simulink model "Lab1"  (R2023b)
settings: Solver=VariableStepAuto  StartTime=0.0  StopTime=10  RelTol=1e-3
undefined symbols (not defined in the file): sigbuilder_block
libraries: fl_lib x35, sh_lib x22, nesl_utility x20
settings Model: Creator=agluh  LastModifiedBy=a2
settings SolverCC: AlgebraicLoopSolver=TrustRegion
settings ModelReferenceCC: EnableRefExpFcnMdlSchedulingChecks=on
settings SimscapeCC: ExplicitSolverDiagnosticOptions=none

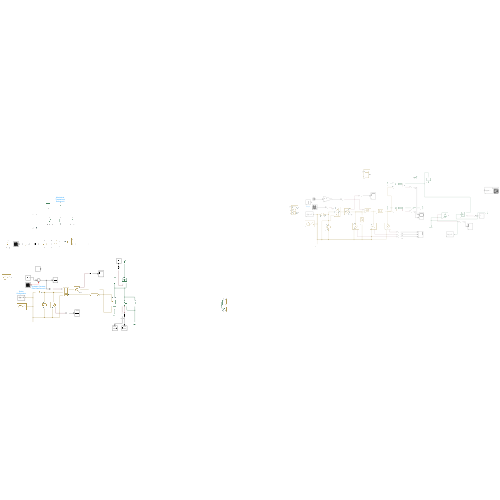
[thumbnail: Simulink's stored preview of the top-level diagram]
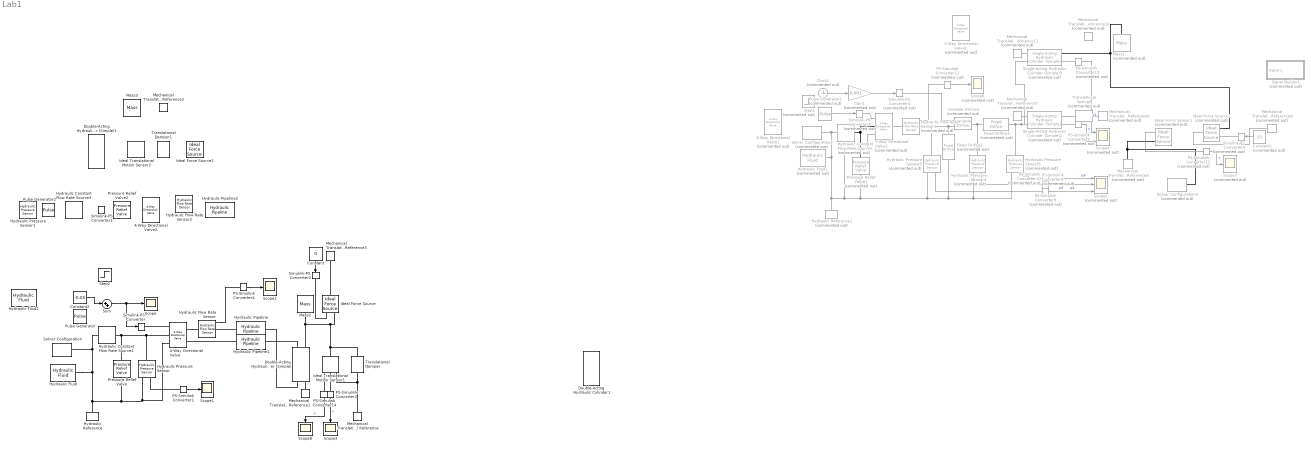
== system Lab1 ==
  2-Way Directional Valve2 : sh_lib/Valves/Directional Valves/2-Way Directional Valve  Commented=on  mdl_type=1  area_max=0.1 m^2  opening_max=0.1 m  opening_tab=[-.002, 0, .002, .005, .015] m  area_tab=[1e-09, 2.0352e-07, 4.0736e-05, .00011438, .00034356] m^2  pressure_tab=[-10000000, -5000000, -2000000, 2000000, 5000000, 10000000] Pa  flow_rate_tab=[-1e-07, -7.0711e-08, -4.4721e-08, 4.4721e-08, 7.0711e-08, 1e-07; -2.0352e-05, -1.4391e-05, -9.1017e-06, 9.1017e-06, 1.4391e-05, 2.0352e-05; -.0040736, -.0028805, -.0018218, .0018218, .0028805, .0040736; -.011438, -.0080879, -.0051152, .0051152, .0080879, .011438; -.034356, -.024293, -.015364, .015364, .024293, .034356] m^3/s  interp_method=1  extrap_method=1  C_d=0.7  x_0=0 m  A_leak=1e-12 m^2  lam_spec=1  B_lam=0.999  Re_cr=12
      settings: InternalSimscapePortConfiguration="{\"Bottom\":[],\"Left\":[{\"id\":\"S\",\"label\":\"S\",\"type\":\"input\"},{\"id\":\"A\",\"label\":\"A\",\"type\":\"foundation.hydraulic.hydraulic\"}],\"Right\":[{\"id\":\"B\",\"label\":\"B\",\"type\":\"foundation.hydraulic.hydraulic\"}],\"Top\":[]}"
  3-Way Directional Valve1 : sh_lib/Valves/Directional Valves/3-Way Directional Valve  Commented=on  area_spec=sh.valves.directional_valves.enum.area_spec.identical  mdl_type_identical=sh.valves.directional_valves.enum.mdl_type.linear  mdl_type_different=sh.valves.directional_valves.enum.mdl_type.linear  interp_method_identical=sh.valves.directional_valves.enum.interp_method.linear  interp_method_different=sh.valves.directional_valves.enum.interp_method.linear  extrap_method_identical=sh.valves.directional_valves.enum.extrap_method.linear  extrap_method_different=sh.valves.directional_valves.enum.extrap_method.linear  A_leak=0.0000000000001 mm^2  C_d=0.7  lam_spec=sh.valves.directional_valves.enum.lam_spec.pressure_ratio  B_lam=0.999  Re_cr=12  opening_max=0.1 m  area_max=0.1 m^2  opening_max_P_A=0.005 m  area_max_P_A=0.5e-4 m^2  opening_max_A_T=0.005 m  area_max_A_T=0.5e-4 m^2  opening_area_tab=[-.002, 0, .002, .005, .015] m  area_tab=[1e-09, 2.0352e-07, 4.0736e-05, .00011438, .00034356] m^2  opening_flow_rate_tab=[-.002, 0, .002, .005, .015] m  pressure_tab=[-10000000, -5000000, -2000000, 2000000, 5000000, 10000000] Pa  flow_rate_tab=[-1e-07, -7.0711e-08, -4.4721e-08, 4.4721e-08, 7.0711e-08, 1e-07; -2.0352e-05, -1.4391e-05, -9.1017e-06, 9.1017e-06, 1.4391e-05, 2.0352e-05; -.0040736, -.0028805, -.0018218, .0018218, .0028805, .0040736; -.011438, -.0080879, -.0051152, .0051152, .0080879, .011438; -.034356, -.024293, -.015364, .015364, .024293, .034356] m^3/s  opening_area_tab_P_A=[-.002, 0, .002, .005, .015] m  area_tab_P_A=[1e-09, 2.0352e-07, 4.0736e-05, .00011438, .00034356] m^2  opening_flow_rate_tab_P_A=[-.002, 0, .002, .005, .015] m  pressure_tab_P_A=[-10000000, -5000000, -2000000, 2000000, 5000000, 10000000] Pa  flow_rate_tab_P_A=[-1e-07, -7.0711e-08, -4.4721e-08, 4.4721e-08, 7.0711e-08, 1e-07; -2.0352e-05, -1.4391e-05, -9.1017e-06, 9.1017e-06, 1.4391e-05, 2.0352e-05; -.0040736, -.0028805, -.0018218, .0018218, .0028805, .0040736; -.011438, -.0080879, -.0051152, .0051152, .0080879, .011438; -.034356, -.024293, -.015364, .015364, .024293, .034356] m^3/s  opening_area_tab_A_T=[-.002, 0, .002, .005, .015] m  area_tab_A_T=[1e-09, 2.0352e-07, 4.0736e-05, .00011438, .00034356] m^2  opening_flow_rate_tab_A_T=[-.002, 0, .002, .005, .015] m  pressure_tab_A_T=[-10000000, -5000000, -2000000, 2000000, 5000000, 10000000] Pa  flow_rate_tab_A_T=[-1e-07, -7.0711e-08, -4.4721e-08, 4.4721e-08, 7.0711e-08, 1e-07; -2.0352e-05, -1.4391e-05, -9.1017e-06, 9.1017e-06, 1.4391e-05, 2.0352e-05; -.0040736, -.0028805, -.0018218, .0018218, .0028805, .0040736; -.011438, -.0080879, -.0051152, .0051152, .0080879, .011438; -.034356, -.024293, -.015364, .015364, .024293, .034356] m^3/s  x_0_P=0.1 m  x_0_T=0.1 m
      settings: InternalSimscapePortConfiguration="{\"Bottom\":[],\"Left\":[{\"id\":\"A\",\"label\":\"A\",\"type\":\"foundation.hydraulic.hydraulic\"}],\"Right\":[{\"id\":\"S\",\"label\":\"S\",\"type\":\"input\"},{\"id\":\"P\",\"label\":\"P\",\"type\":\"foundation.hydraulic.hydraulic\"},{\"id\":\"T\",\"label\":\"T\",\"type\":\"foundation.hydraulic.hydraulic\"}],\"Top\":[]}"
  4-Way Directional Valve : sh_lib/Valves/Directional Valves/4-Way Directional Valve  area_spec=sh.valves.directional_valves.enum.area_spec.identical  mdl_type_identical=sh.valves.directional_valves.enum.mdl_type.linear  mdl_type_different=sh.valves.directional_valves.enum.mdl_type.linear  interp_method_identical=sh.valves.directional_valves.enum.interp_method.linear  interp_method_different=sh.valves.directional_valves.enum.interp_method.linear  extrap_method_identical=sh.valves.directional_valves.enum.extrap_method.linear  extrap_method_different=sh.valves.directional_valves.enum.extrap_method.linear  A_leak=1e-12 m^2  C_d=0.7  lam_spec=sh.valves.directional_valves.enum.lam_spec.pressure_ratio  B_lam=0.999  Re_cr=12  opening_max=0.01 m  area_max=0.5e-5 m^2  opening_max_P_A=0.005 m  area_max_P_A=0.5e-4 m^2  opening_max_P_B=0.005 m  area_max_P_B=0.5e-4 m^2  opening_max_A_T=0.005 m  area_max_A_T=0.5e-4 m^2  opening_max_B_T=0.005 m  area_max_B_T=0.5e-4 m^2  opening_area_tab=[-.002, 0, .002, .005, .015] m  area_tab=[1e-09, 2.0352e-07, 4.0736e-05, .00011438, .00034356] m^2  opening_flow_rate_tab=[-.002, 0, .002, .005, .015] m  pressure_tab=[-10000000, -5000000, -2000000, 2000000, 5000000, 10000000] Pa  flow_rate_tab=[-1e-07, -7.0711e-08, -4.4721e-08, 4.4721e-08, 7.0711e-08, 1e-07; -2.0352e-05, -1.4391e-05, -9.1017e-06, 9.1017e-06, 1.4391e-05, 2.0352e-05; -.0040736, -.0028805, -.0018218, .0018218, .0028805, .0040736; -.011438, -.0080879, -.0051152, .0051152, .0080879, .011438; -.034356, -.024293, -.015364, .015364, .024293, .034356] m^3/s  opening_area_tab_P_A=[-.002, 0, .002, .005, .015] m  area_tab_P_A=[1e-09, 2.0352e-07, 4.0736e-05, .00011438, .00034356] m^2  opening_flow_rate_tab_P_A=[-.002, 0, .002, .005, .015] m  pressure_tab_P_A=[-10000000, -5000000, -2000000, 2000000, 5000000, 10000000] Pa  flow_rate_tab_P_A=[-1e-07, -7.0711e-08, -4.4721e-08, 4.4721e-08, 7.0711e-08, 1e-07; -2.0352e-05, -1.4391e-05, -9.1017e-06, 9.1017e-06, 1.4391e-05, 2.0352e-05; -.0040736, -.0028805, -.0018218, .0018218, .0028805, .0040736; -.011438, -.0080879, -.0051152, .0051152, .0080879, .011438; -.034356, -.024293, -.015364, .015364, .024293, .034356] m^3/s  opening_area_tab_P_B=[-.002, 0, .002, .005, .015] m  area_tab_P_B=[1e-09, 2.0352e-07, 4.0736e-05, .00011438, .00034356] m^2  opening_flow_rate_tab_P_B=[-.002, 0, .002, .005, .015] m  pressure_tab_P_B=[-10000000, -5000000, -2000000, 2000000, 5000000, 10000000] Pa  flow_rate_tab_P_B=[-1e-07, -7.0711e-08, -4.4721e-08, 4.4721e-08, 7.0711e-08, 1e-07; -2.0352e-05, -1.4391e-05, -9.1017e-06, 9.1017e-06, 1.4391e-05, 2.0352e-05; -.0040736, -.0028805, -.0018218, .0018218, .0028805, .0040736; -.011438, -.0080879, -.0051152, .0051152, .0080879, .011438; -.034356, -.024293, -.015364, .015364, .024293, .034356] m^3/s  opening_area_tab_A_T=[-.002, 0, .002, .005, .015] m  area_tab_A_T=[1e-09, 2.0352e-07, 4.0736e-05, .00011438, .00034356] m^2  opening_flow_rate_tab_A_T=[-.002, 0, .002, .005, .015] m  pressure_tab_A_T=[-10000000, -5000000, -2000000, 2000000, 5000000, 10000000] Pa  flow_rate_tab_A_T=[-1e-07, -7.0711e-08, -4.4721e-08, 4.4721e-08, 7.0711e-08, 1e-07; -2.0352e-05, -1.4391e-05, -9.1017e-06, 9.1017e-06, 1.4391e-05, 2.0352e-05; -.0040736, -.0028805, -.0018218, .0018218, .0028805, .0040736; -.011438, -.0080879, -.0051152, .0051152, .0080879, .011438; -.034356, -.024293, -.015364, .015364, .024293, .034356] m^3/s  opening_area_tab_B_T=[-.002, 0, .002, .005, .015] m  area_tab_B_T=[1e-09, 2.0352e-07, 4.0736e-05, .00011438, .00034356] m^2  opening_flow_rate_tab_B_T=[-.002, 0, .002, .005, .015] m  pressure_tab_B_T=[-10000000, -5000000, -2000000, 2000000, 5000000, 10000000] Pa  flow_rate_tab_B_T=[-1e-07, -7.0711e-08, -4.4721e-08, 4.4721e-08, 7.0711e-08, 1e-07; -2.0352e-05, -1.4391e-05, -9.1017e-06, 9.1017e-06, 1.4391e-05, 2.0352e-05; -.0040736, -.0028805, -.0018218, .0018218, .0028805, .0040736; -.011438, -.0080879, -.0051152, .0051152, .0080879, .011438; -.034356, -.024293, -.015364, .015364, .024293, .034356] m^3/s  x_0_P_A=0 m  x_0_P_B=0 m  x_0_A_T=0 m  x_0_B_T=0 m
      settings: InternalSimscapePortConfiguration="{\"Bottom\":[],\"Left\":[{\"id\":\"A\",\"label\":\"A\",\"type\":\"foundation.hydraulic.hydraulic\"},{\"id\":\"B\",\"label\":\"B\",\"type\":\"foundation.hydraulic.hydraulic\"}],\"Right\":[{\"id\":\"S\",\"label\":\"S\",\"type\":\"input\"},{\"id\":\"P\",\"label\":\"P\",\"type\":\"foundation.hydraulic.hydraulic\"},{\"id\":\"T\",\"label\":\"T\",\"type\":\"foundation.hydraulic.hydraulic\"}],\"Top\":[]}"
  4-Way Directional Valve1 : sh_lib/Valves/Directional Valves/4-Way Directional Valve  Commented=on  area_spec=sh.valves.directional_valves.enum.area_spec.identical  mdl_type_identical=sh.valves.directional_valves.enum.mdl_type.linear  mdl_type_different=sh.valves.directional_valves.enum.mdl_type.linear  interp_method_identical=sh.valves.directional_valves.enum.interp_method.linear  interp_method_different=sh.valves.directional_valves.enum.interp_method.linear  extrap_method_identical=sh.valves.directional_valves.enum.extrap_method.linear  extrap_method_different=sh.valves.directional_valves.enum.extrap_method.linear  A_leak=1e-12 m^2  C_d=0.7  lam_spec=sh.valves.directional_valves.enum.lam_spec.pressure_ratio  B_lam=0.999  Re_cr=12  opening_max=0.005 m  area_max=0.5e-4 m^2  opening_max_P_A=0.005 m  area_max_P_A=0.5e-4 m^2  opening_max_P_B=0.005 m  area_max_P_B=0.5e-4 m^2  opening_max_A_T=0.005 m  area_max_A_T=0.5e-4 m^2  opening_max_B_T=0.005 m  area_max_B_T=0.5e-4 m^2  opening_area_tab=[-.002, 0, .002, .005, .015] m  area_tab=[1e-09, 2.0352e-07, 4.0736e-05, .00011438, .00034356] m^2  opening_flow_rate_tab=[-.002, 0, .002, .005, .015] m  pressure_tab=[-10000000, -5000000, -2000000, 2000000, 5000000, 10000000] Pa  flow_rate_tab=[-1e-07, -7.0711e-08, -4.4721e-08, 4.4721e-08, 7.0711e-08, 1e-07; -2.0352e-05, -1.4391e-05, -9.1017e-06, 9.1017e-06, 1.4391e-05, 2.0352e-05; -.0040736, -.0028805, -.0018218, .0018218, .0028805, .0040736; -.011438, -.0080879, -.0051152, .0051152, .0080879, .011438; -.034356, -.024293, -.015364, .015364, .024293, .034356] m^3/s  opening_area_tab_P_A=[-.002, 0, .002, .005, .015] m  area_tab_P_A=[1e-09, 2.0352e-07, 4.0736e-05, .00011438, .00034356] m^2  opening_flow_rate_tab_P_A=[-.002, 0, .002, .005, .015] m  pressure_tab_P_A=[-10000000, -5000000, -2000000, 2000000, 5000000, 10000000] Pa  flow_rate_tab_P_A=[-1e-07, -7.0711e-08, -4.4721e-08, 4.4721e-08, 7.0711e-08, 1e-07; -2.0352e-05, -1.4391e-05, -9.1017e-06, 9.1017e-06, 1.4391e-05, 2.0352e-05; -.0040736, -.0028805, -.0018218, .0018218, .0028805, .0040736; -.011438, -.0080879, -.0051152, .0051152, .0080879, .011438; -.034356, -.024293, -.015364, .015364, .024293, .034356] m^3/s  opening_area_tab_P_B=[-.002, 0, .002, .005, .015] m  area_tab_P_B=[1e-09, 2.0352e-07, 4.0736e-05, .00011438, .00034356] m^2  opening_flow_rate_tab_P_B=[-.002, 0, .002, .005, .015] m  pressure_tab_P_B=[-10000000, -5000000, -2000000, 2000000, 5000000, 10000000] Pa  flow_rate_tab_P_B=[-1e-07, -7.0711e-08, -4.4721e-08, 4.4721e-08, 7.0711e-08, 1e-07; -2.0352e-05, -1.4391e-05, -9.1017e-06, 9.1017e-06, 1.4391e-05, 2.0352e-05; -.0040736, -.0028805, -.0018218, .0018218, .0028805, .0040736; -.011438, -.0080879, -.0051152, .0051152, .0080879, .011438; -.034356, -.024293, -.015364, .015364, .024293, .034356] m^3/s  opening_area_tab_A_T=[-.002, 0, .002, .005, .015] m  area_tab_A_T=[1e-09, 2.0352e-07, 4.0736e-05, .00011438, .00034356] m^2  opening_flow_rate_tab_A_T=[-.002, 0, .002, .005, .015] m  pressure_tab_A_T=[-10000000, -5000000, -2000000, 2000000, 5000000, 10000000] Pa  flow_rate_tab_A_T=[-1e-07, -7.0711e-08, -4.4721e-08, 4.4721e-08, 7.0711e-08, 1e-07; -2.0352e-05, -1.4391e-05, -9.1017e-06, 9.1017e-06, 1.4391e-05, 2.0352e-05; -.0040736, -.0028805, -.0018218, .0018218, .0028805, .0040736; -.011438, -.0080879, -.0051152, .0051152, .0080879, .011438; -.034356, -.024293, -.015364, .015364, .024293, .034356] m^3/s  opening_area_tab_B_T=[-.002, 0, .002, .005, .015] m  area_tab_B_T=[1e-09, 2.0352e-07, 4.0736e-05, .00011438, .00034356] m^2  opening_flow_rate_tab_B_T=[-.002, 0, .002, .005, .015] m  pressure_tab_B_T=[-10000000, -5000000, -2000000, 2000000, 5000000, 10000000] Pa  flow_rate_tab_B_T=[-1e-07, -7.0711e-08, -4.4721e-08, 4.4721e-08, 7.0711e-08, 1e-07; -2.0352e-05, -1.4391e-05, -9.1017e-06, 9.1017e-06, 1.4391e-05, 2.0352e-05; -.0040736, -.0028805, -.0018218, .0018218, .0028805, .0040736; -.011438, -.0080879, -.0051152, .0051152, .0080879, .011438; -.034356, -.024293, -.015364, .015364, .024293, .034356] m^3/s  x_0_P_A=0 m  x_0_P_B=0 m  x_0_A_T=0 m  x_0_B_T=0 m
      settings: InternalSimscapePortConfiguration="{\"Bottom\":[],\"Left\":[{\"id\":\"A\",\"label\":\"A\",\"type\":\"foundation.hydraulic.hydraulic\"},{\"id\":\"B\",\"label\":\"B\",\"type\":\"foundation.hydraulic.hydraulic\"}],\"Right\":[{\"id\":\"S\",\"label\":\"S\",\"type\":\"input\"},{\"id\":\"P\",\"label\":\"P\",\"type\":\"foundation.hydraulic.hydraulic\"},{\"id\":\"T\",\"label\":\"T\",\"type\":\"foundation.hydraulic.hydraulic\"}],\"Top\":[]}"
  4-Way Directional Valve2 : sh_lib/Valves/Directional Valves/4-Way Directional Valve  area_spec=sh.valves.directional_valves.enum.area_spec.identical  mdl_type_identical=sh.valves.directional_valves.enum.mdl_type.linear  mdl_type_different=sh.valves.directional_valves.enum.mdl_type.linear  interp_method_identical=sh.valves.directional_valves.enum.interp_method.linear  interp_method_different=sh.valves.directional_valves.enum.interp_method.linear  extrap_method_identical=sh.valves.directional_valves.enum.extrap_method.linear  extrap_method_different=sh.valves.directional_valves.enum.extrap_method.linear  A_leak=1e-12 m^2  C_d=0.7  lam_spec=sh.valves.directional_valves.enum.lam_spec.pressure_ratio  B_lam=0.999  Re_cr=12  opening_max=0.01 m  area_max=0.5e-5 m^2  opening_max_P_A=0.005 m  area_max_P_A=0.5e-4 m^2  opening_max_P_B=0.005 m  area_max_P_B=0.5e-4 m^2  opening_max_A_T=0.005 m  area_max_A_T=0.5e-4 m^2  opening_max_B_T=0.005 m  area_max_B_T=0.5e-4 m^2  opening_area_tab=[-.002, 0, .002, .005, .015] m  area_tab=[1e-09, 2.0352e-07, 4.0736e-05, .00011438, .00034356] m^2  opening_flow_rate_tab=[-.002, 0, .002, .005, .015] m  pressure_tab=[-10000000, -5000000, -2000000, 2000000, 5000000, 10000000] Pa  flow_rate_tab=[-1e-07, -7.0711e-08, -4.4721e-08, 4.4721e-08, 7.0711e-08, 1e-07; -2.0352e-05, -1.4391e-05, -9.1017e-06, 9.1017e-06, 1.4391e-05, 2.0352e-05; -.0040736, -.0028805, -.0018218, .0018218, .0028805, .0040736; -.011438, -.0080879, -.0051152, .0051152, .0080879, .011438; -.034356, -.024293, -.015364, .015364, .024293, .034356] m^3/s  opening_area_tab_P_A=[-.002, 0, .002, .005, .015] m  area_tab_P_A=[1e-09, 2.0352e-07, 4.0736e-05, .00011438, .00034356] m^2  opening_flow_rate_tab_P_A=[-.002, 0, .002, .005, .015] m  pressure_tab_P_A=[-10000000, -5000000, -2000000, 2000000, 5000000, 10000000] Pa  flow_rate_tab_P_A=[-1e-07, -7.0711e-08, -4.4721e-08, 4.4721e-08, 7.0711e-08, 1e-07; -2.0352e-05, -1.4391e-05, -9.1017e-06, 9.1017e-06, 1.4391e-05, 2.0352e-05; -.0040736, -.0028805, -.0018218, .0018218, .0028805, .0040736; -.011438, -.0080879, -.0051152, .0051152, .0080879, .011438; -.034356, -.024293, -.015364, .015364, .024293, .034356] m^3/s  opening_area_tab_P_B=[-.002, 0, .002, .005, .015] m  area_tab_P_B=[1e-09, 2.0352e-07, 4.0736e-05, .00011438, .00034356] m^2  opening_flow_rate_tab_P_B=[-.002, 0, .002, .005, .015] m  pressure_tab_P_B=[-10000000, -5000000, -2000000, 2000000, 5000000, 10000000] Pa  flow_rate_tab_P_B=[-1e-07, -7.0711e-08, -4.4721e-08, 4.4721e-08, 7.0711e-08, 1e-07; -2.0352e-05, -1.4391e-05, -9.1017e-06, 9.1017e-06, 1.4391e-05, 2.0352e-05; -.0040736, -.0028805, -.0018218, .0018218, .0028805, .0040736; -.011438, -.0080879, -.0051152, .0051152, .0080879, .011438; -.034356, -.024293, -.015364, .015364, .024293, .034356] m^3/s  opening_area_tab_A_T=[-.002, 0, .002, .005, .015] m  area_tab_A_T=[1e-09, 2.0352e-07, 4.0736e-05, .00011438, .00034356] m^2  opening_flow_rate_tab_A_T=[-.002, 0, .002, .005, .015] m  pressure_tab_A_T=[-10000000, -5000000, -2000000, 2000000, 5000000, 10000000] Pa  flow_rate_tab_A_T=[-1e-07, -7.0711e-08, -4.4721e-08, 4.4721e-08, 7.0711e-08, 1e-07; -2.0352e-05, -1.4391e-05, -9.1017e-06, 9.1017e-06, 1.4391e-05, 2.0352e-05; -.0040736, -.0028805, -.0018218, .0018218, .0028805, .0040736; -.011438, -.0080879, -.0051152, .0051152, .0080879, .011438; -.034356, -.024293, -.015364, .015364, .024293, .034356] m^3/s  opening_area_tab_B_T=[-.002, 0, .002, .005, .015] m  area_tab_B_T=[1e-09, 2.0352e-07, 4.0736e-05, .00011438, .00034356] m^2  opening_flow_rate_tab_B_T=[-.002, 0, .002, .005, .015] m  pressure_tab_B_T=[-10000000, -5000000, -2000000, 2000000, 5000000, 10000000] Pa  flow_rate_tab_B_T=[-1e-07, -7.0711e-08, -4.4721e-08, 4.4721e-08, 7.0711e-08, 1e-07; -2.0352e-05, -1.4391e-05, -9.1017e-06, 9.1017e-06, 1.4391e-05, 2.0352e-05; -.0040736, -.0028805, -.0018218, .0018218, .0028805, .0040736; -.011438, -.0080879, -.0051152, .0051152, .0080879, .011438; -.034356, -.024293, -.015364, .015364, .024293, .034356] m^3/s  x_0_P_A=0 m  x_0_P_B=0 m  x_0_A_T=0 m  x_0_B_T=0 m
      settings: InternalSimscapePortConfiguration="{\"Bottom\":[],\"Left\":[{\"id\":\"A\",\"label\":\"A\",\"type\":\"foundation.hydraulic.hydraulic\"},{\"id\":\"B\",\"label\":\"B\",\"type\":\"foundation.hydraulic.hydraulic\"}],\"Right\":[{\"id\":\"S\",\"label\":\"S\",\"type\":\"input\"},{\"id\":\"P\",\"label\":\"P\",\"type\":\"foundation.hydraulic.hydraulic\"},{\"id\":\"T\",\"label\":\"T\",\"type\":\"foundation.hydraulic.hydraulic\"}],\"Top\":[]}"
  Clock1 : Clock  Commented=on
  Constant : Constant  Value=0
  Constant1 : Constant  Commented=on  Value=10
  Constant2 : Constant  Value=-0.05
  Double-Acting Hydraulic Cylinder (Simple) : sh_lib/Hydraulic Cylinders/Double-Acting Hydraulic Cylinder (Simple)  area_A=1e-3 m^2  area_B=1e-3 m^2  stroke=0.5 m  init_pos=0 m  penetr_coeff=1e12 N*s/m^2  or=1
      settings: InternalSimscapePortConfiguration="{\"Bottom\":[],\"Left\":[{\"id\":\"C\",\"label\":\"C\",\"type\":\"foundation.mechanical.translational.translational\"},{\"id\":\"A\",\"label\":\"A\",\"type\":\"foundation.hydraulic.hydraulic\"}],\"Right\":[{\"id\":\"R\",\"label\":\"R\",\"type\":\"foundation.mechanical.translational.translational\"},{\"id\":\"B\",\"label\":\"B\",\"type\":\"foundation.hydraulic.hydraulic\"}],\"Top\":[]}"
  Double-Acting Hydraulic Cylinder (Simple)1 : sh_lib/Hydraulic Cylinders/Double-Acting Hydraulic Cylinder (Simple)  area_A=1e-3 m^2  area_B=1e-3 m^2  stroke=0.5 m  init_pos=0 m  penetr_coeff=1e12 N*s/m^2  or=1
      settings: InternalSimscapePortConfiguration="{\"Bottom\":[],\"Left\":[{\"id\":\"C\",\"label\":\"C\",\"type\":\"foundation.mechanical.translational.translational\"},{\"id\":\"A\",\"label\":\"A\",\"type\":\"foundation.hydraulic.hydraulic\"}],\"Right\":[{\"id\":\"R\",\"label\":\"R\",\"type\":\"foundation.mechanical.translational.translational\"},{\"id\":\"B\",\"label\":\"B\",\"type\":\"foundation.hydraulic.hydraulic\"}],\"Top\":[]}"
  Double-Acting Hydraulic Cylinder1 : sh_lib/Hydraulic Cylinders/Double-Acting Hydraulic Cylinder  area_A=0.01 m^2  area_B=0.01 m^2  stroke=2 m  dead_vol_A=1e-4 m^3  dead_vol_B=1e-4 m^3  k_sh=1.4  or=1  stiff=1e8 N/m  D=150 N/(m/s)  hardstop_model=1  transition=0.1 mm  displacement_spec=foundation.enum.DisplacementSpec.Calculate  init_pos=0.1 m  init_pressure_A=0 Pa  init_pressure_B=0 Pa
      settings: InternalSimscapePortConfiguration="{\"Bottom\":[],\"Left\":[{\"id\":\"C\",\"label\":\"C\",\"type\":\"foundation.mechanical.translational.translational\"},{\"id\":\"A\",\"label\":\"A\",\"type\":\"foundation.hydraulic.hydraulic\"}],\"Right\":[{\"id\":\"R\",\"label\":\"R\",\"type\":\"foundation.mechanical.translational.translational\"},{\"id\":\"B\",\"label\":\"B\",\"type\":\"foundation.hydraulic.hydraulic\"}],\"Top\":[]}"
  Fixed Orifice2 : sh_lib/Orifices/Fixed Orifice  Commented=on  area=1e-4 m^2  C_d=0.7  lam_spec=1  B_lam=2E-8  Re_cr=12  q_specify=off  q_priority=None  q=1e-3 m^3/s  q_nominal_specify=off  q_nominal_unit=m^3/s  q_nominal_value=1  p_specify=off  p_priority=None  p=0 Pa  p_nominal_specify=off  p_nominal_unit=Pa  p_nominal_value=1
      settings: InternalSimscapePortConfiguration="{\"Bottom\":[],\"Left\":[{\"id\":\"A\",\"label\":\"A\",\"type\":\"foundation.hydraulic.hydraulic\"}],\"Right\":[{\"id\":\"B\",\"label\":\"B\",\"type\":\"foundation.hydraulic.hydraulic\"}],\"Top\":[]}"
  Fixed Orifice3 : sh_lib/Orifices/Fixed Orifice  Commented=on  area=1e-4 m^2  C_d=0.7  lam_spec=1  B_lam=2E-8  Re_cr=12  q_specify=off  q_priority=None  q=1e-3 m^3/s  q_nominal_specify=off  q_nominal_unit=m^3/s  q_nominal_value=1  p_specify=off  p_priority=None  p=0 Pa  p_nominal_specify=off  p_nominal_unit=Pa  p_nominal_value=1
      settings: InternalSimscapePortConfiguration="{\"Bottom\":[],\"Left\":[{\"id\":\"A\",\"label\":\"A\",\"type\":\"foundation.hydraulic.hydraulic\"}],\"Right\":[{\"id\":\"B\",\"label\":\"B\",\"type\":\"foundation.hydraulic.hydraulic\"}],\"Top\":[]}"
  Gain1 : Gain  Commented=on  Gain=0.001  SaturateOnIntegerOverflow=on  OutDataTypeStr=Inherit: Same as input  ParamDataTypeStr=Inherit: Same as input
  Hydraulic Constant Flow Rate Source1 : fl_lib/Hydraulic/Hydraulic Sources/Hydraulic Constant Flow Rate Source  Commented=on  commanded_flow_rate=0.005 m^3/s
      settings: InternalSimscapePortConfiguration="{\"Bottom\":[],\"Left\":[{\"id\":\"P\",\"label\":\"P\",\"type\":\"foundation.hydraulic.hydraulic\"}],\"Right\":[{\"id\":\"T\",\"label\":\"T\",\"type\":\"foundation.hydraulic.hydraulic\"}],\"Top\":[]}"
  Hydraulic Constant Flow Rate Source2 : fl_lib/Hydraulic/Hydraulic Sources/Hydraulic Constant Flow Rate Source  commanded_flow_rate=0.007 m^3/s
      settings: InternalSimscapePortConfiguration="{\"Bottom\":[],\"Left\":[{\"id\":\"P\",\"label\":\"P\",\"type\":\"foundation.hydraulic.hydraulic\"}],\"Right\":[{\"id\":\"T\",\"label\":\"T\",\"type\":\"foundation.hydraulic.hydraulic\"}],\"Top\":[]}"
  Hydraulic Constant Flow Rate Source3 : fl_lib/Hydraulic/Hydraulic Sources/Hydraulic Constant Flow Rate Source  commanded_flow_rate=0.007 m^3/s
      settings: InternalSimscapePortConfiguration="{\"Bottom\":[],\"Left\":[{\"id\":\"P\",\"label\":\"P\",\"type\":\"foundation.hydraulic.hydraulic\"}],\"Right\":[{\"id\":\"T\",\"label\":\"T\",\"type\":\"foundation.hydraulic.hydraulic\"}],\"Top\":[]}"
  Hydraulic Flow Rate Sensor : fl_lib/Hydraulic/Hydraulic Sensors/Hydraulic Flow Rate Sensor
  Hydraulic Flow Rate Sensor1 : fl_lib/Hydraulic/Hydraulic Sensors/Hydraulic Flow Rate Sensor  Commented=on
  Hydraulic Flow Rate Sensor2 : fl_lib/Hydraulic/Hydraulic Sensors/Hydraulic Flow Rate Sensor
  Hydraulic Fluid : sh_lib/Hydraulic Utilities/Hydraulic Fluid  SelFluid=24  SysTemp=60  TrapAir=0.005  ViscDerFactor=1  range_error=2
  Hydraulic Fluid1 : sh_lib/Hydraulic Utilities/Hydraulic Fluid  Commented=on  SelFluid=24  SysTemp=60  TrapAir=0.005  ViscDerFactor=1  range_error=2
  Hydraulic Fluid2 : sh_lib/Hydraulic Utilities/Hydraulic Fluid  SelFluid=1  SysTemp=60  TrapAir=0.005  ViscDerFactor=1  range_error=2
  Hydraulic Pipeline : sh_lib/Pipelines/Hydraulic Pipeline  cs_type=foundation.enum.pipeCrossSection.circular  d_in=1 cm  area=1e-4 m^2  D_h=1.12e-2 m  s_factor=64  length=100 cm  length_ad=1 m  roughness=15e-6 m  Re_lam=2000  Re_turb=4000  wall_type=foundation.enum.chamber_spec.rigid  pr_r_coef=2e-12 m/Pa  time_const=0.01 s  k_sh=1.4  initial_pressure=1 Pa
      settings: InternalSimscapePortConfiguration="{\"Bottom\":[],\"Left\":[{\"id\":\"A\",\"label\":\"A\",\"type\":\"foundation.hydraulic.hydraulic\"}],\"Right\":[{\"id\":\"B\",\"label\":\"B\",\"type\":\"foundation.hydraulic.hydraulic\"}],\"Top\":[]}"
  Hydraulic Pipeline1 : sh_lib/Pipelines/Hydraulic Pipeline  cs_type=foundation.enum.pipeCrossSection.circular  d_in=1 cm  area=1e-4 m^2  D_h=1.12e-2 m  s_factor=64  length=100 cm  length_ad=1 m  roughness=15e-6 m  Re_lam=2000  Re_turb=4000  wall_type=foundation.enum.chamber_spec.rigid  pr_r_coef=2e-12 m/Pa  time_const=0.01 s  k_sh=1.4  initial_pressure=1 Pa
      settings: InternalSimscapePortConfiguration="{\"Bottom\":[],\"Left\":[{\"id\":\"A\",\"label\":\"A\",\"type\":\"foundation.hydraulic.hydraulic\"}],\"Right\":[{\"id\":\"B\",\"label\":\"B\",\"type\":\"foundation.hydraulic.hydraulic\"}],\"Top\":[]}"
  Hydraulic Pipeline2 : sh_lib/Pipelines/Hydraulic Pipeline  cs_type=foundation.enum.pipeCrossSection.circular  d_in=1 cm  area=1e-4 m^2  D_h=1.12e-2 m  s_factor=64  length=100 cm  length_ad=1 m  roughness=15e-6 m  Re_lam=2000  Re_turb=4000  wall_type=foundation.enum.chamber_spec.rigid  pr_r_coef=2e-12 m/Pa  time_const=0.01 s  k_sh=1.4  initial_pressure=1 Pa
      settings: InternalSimscapePortConfiguration="{\"Bottom\":[],\"Left\":[{\"id\":\"A\",\"label\":\"A\",\"type\":\"foundation.hydraulic.hydraulic\"}],\"Right\":[{\"id\":\"B\",\"label\":\"B\",\"type\":\"foundation.hydraulic.hydraulic\"}],\"Top\":[]}"
  Hydraulic Pressure Sensor : fl_lib/Hydraulic/Hydraulic Sensors/Hydraulic Pressure Sensor
  Hydraulic Pressure Sensor1 : fl_lib/Hydraulic/Hydraulic Sensors/Hydraulic Pressure Sensor
  Hydraulic Pressure Sensor3 : fl_lib/Hydraulic/Hydraulic Sensors/Hydraulic Pressure Sensor  Commented=on
  Hydraulic Pressure Sensor4 : fl_lib/Hydraulic/Hydraulic Sensors/Hydraulic Pressure Sensor  Commented=on
  Hydraulic Pressure Sensor5 : fl_lib/Hydraulic/Hydraulic Sensors/Hydraulic Pressure Sensor  Commented=on
  Hydraulic Reference : fl_lib/Hydraulic/Hydraulic Elements/Hydraulic Reference
  Hydraulic Reference1 : fl_lib/Hydraulic/Hydraulic Elements/Hydraulic Reference  Commented=on
  Ideal Force Sensor1 : fl_lib/Mechanical/Mechanical Sensors/Ideal Force Sensor  Commented=on
  Ideal Force Source : fl_lib/Mechanical/Mechanical Sources/Ideal Force Source
  Ideal Force Source1 : fl_lib/Mechanical/Mechanical Sources/Ideal Force Source  Commented=on
  Ideal Force Source2 : fl_lib/Mechanical/Mechanical Sources/Ideal Force Source
  Ideal Translational Motion Sensor1 : fl_lib/Mechanical/Mechanical Sensors/Ideal Translational Motion Sensor  reference=foundation.enum.MeasurementReference.difference  acceleration_port=false  velocity_port=true  position_port=true  offset=0 m
  Ideal Translational Motion Sensor2 : fl_lib/Mechanical/Mechanical Sensors/Ideal Translational Motion Sensor  reference=foundation.enum.MeasurementReference.difference  acceleration_port=false  velocity_port=true  position_port=true  offset=0 m
  Mass1 : fl_lib/Mechanical/Translational Elements/Mass  Commented=on  mass=10 kg  num_ports=foundation.enum.numPorts2.one  v_specify=off  v_priority=High  v=0 m/s  v_nominal_specify=off  v_nominal_unit=m/s  v_nominal_value=1  f_specify=off  f_priority=None  f=0 N  f_nominal_specify=off  f_nominal_unit=N  f_nominal_value=1
  Mass2 : fl_lib/Mechanical/Translational Elements/Mass  mass=1000 kg  num_ports=foundation.enum.numPorts2.one  v_specify=off  v_priority=High  v=0 m/s  v_nominal_specify=off  v_nominal_unit=m/s  v_nominal_value=1  f_specify=off  f_priority=None  f=0 N  f_nominal_specify=off  f_nominal_unit=N  f_nominal_value=1
  Mass3 : fl_lib/Mechanical/Translational Elements/Mass  mass=1000 kg  num_ports=foundation.enum.numPorts2.one  v_specify=off  v_priority=High  v=0 m/s  v_nominal_specify=off  v_nominal_unit=m/s  v_nominal_value=1  f_specify=off  f_priority=None  f=0 N  f_nominal_specify=off  f_nominal_unit=N  f_nominal_value=1
  Mechanical Translational Reference{,1..3} (4 alike) : fl_lib/Mechanical/Translational Elements/Mechanical Translational Reference
  Mechanical Translational Reference{6..11} (6 alike) : fl_lib/Mechanical/Translational Elements/Mechanical Translational Reference  Commented=on
  PS-Simulink Converter{1..2,4,14} (4 alike) : nesl_utility/PS-Simulink Converter  PhysicalDomain=network_engine_domain  SubClassName=ps_output  LeftPortType=input  RightPortType=output  PseudoPeriodic=off  Frequencies=[]  VectorFormat=1-D array  Unit=inherit  AffineConversion=off
  PS-Simulink Converter{7..13} (7 alike) : nesl_utility/PS-Simulink Converter  Commented=on  PhysicalDomain=network_engine_domain  SubClassName=ps_output  LeftPortType=input  RightPortType=output  PseudoPeriodic=off  Frequencies=[]  VectorFormat=1-D array  Unit=inherit  AffineConversion=off
  Pressure Relief Valve : sh_lib/Valves/Pressure Control Valves/Pressure Relief Valve  valve_area_spec=1  p_diff_TLU=[30.15e5 : 15e3 : 31.35e5] Pa  area_TLU=[1 : 1 : 9] .* 1e-5 m^2  area_max=0.001 m^2  pres_set=20e6 Pa  reg_range=1 Pa  C_d=0.7  A_leak=1e-12 m^2  lam_spec=1  B_lam=0.999  Re_cr=12  dynamic=0  tau=0.1 s  area_init=1e-12 m^2
      settings: InternalSimscapePortConfiguration="{\"Bottom\":[],\"Left\":[{\"id\":\"A\",\"label\":\"A\",\"type\":\"foundation.hydraulic.hydraulic\"}],\"Right\":[{\"id\":\"B\",\"label\":\"B\",\"type\":\"foundation.hydraulic.hydraulic\"}],\"Top\":[]}"
  Pressure Relief Valve1 : sh_lib/Valves/Pressure Control Valves/Pressure Relief Valve  Commented=on  valve_area_spec=1  p_diff_TLU=[30.15e5 : 15e3 : 31.35e5] Pa  area_TLU=[1 : 1 : 9] .* 1e-5 m^2  area_max=1e-4 m^2  pres_set=20e5 Pa  reg_range=5e5 Pa  C_d=0.7  A_leak=1e-12 m^2  lam_spec=1  B_lam=0.999  Re_cr=12  dynamic=0  tau=0.1 s  area_init=1e-12 m^2
      settings: InternalSimscapePortConfiguration="{\"Bottom\":[],\"Left\":[{\"id\":\"A\",\"label\":\"A\",\"type\":\"foundation.hydraulic.hydraulic\"}],\"Right\":[{\"id\":\"B\",\"label\":\"B\",\"type\":\"foundation.hydraulic.hydraulic\"}],\"Top\":[]}"
  Pressure Relief Valve2 : sh_lib/Valves/Pressure Control Valves/Pressure Relief Valve  valve_area_spec=1  p_diff_TLU=[30.15e5 : 15e3 : 31.35e5] Pa  area_TLU=[1 : 1 : 9] .* 1e-5 m^2  area_max=0.001 m^2  pres_set=20e6 Pa  reg_range=1 Pa  C_d=0.7  A_leak=1e-12 m^2  lam_spec=1  B_lam=0.999  Re_cr=12  dynamic=0  tau=0.1 s  area_init=1e-12 m^2
      settings: InternalSimscapePortConfiguration="{\"Bottom\":[],\"Left\":[{\"id\":\"A\",\"label\":\"A\",\"type\":\"foundation.hydraulic.hydraulic\"}],\"Right\":[{\"id\":\"B\",\"label\":\"B\",\"type\":\"foundation.hydraulic.hydraulic\"}],\"Top\":[]}"
  Pulse Generator : DiscretePulseGenerator  PulseType=Time based  Amplitude=0.1  Period=4  PulseWidth=50
  Pulse Generator1 : DiscretePulseGenerator  Commented=on  PulseType=Time based  Amplitude=0.1  Period=0.025  PulseWidth=50
  Pulse Generator2 : DiscretePulseGenerator  PulseType=Time based  Amplitude=0.1  Period=4  PulseWidth=50
  Scope{,1..3,8} (5 alike) : Scope
  Scope4 : Scope  Commented=on  NumInputPorts=2
  Scope5 : Scope  Commented=on  NumInputPorts=3
  Scope6 : Scope  Commented=on
  Scope7 : Scope  Commented=on
  Signal Builder1 : Subsystem  Tag=STV Subsys  Commented=on  LoadFcn=sigbuilder_block('load');  StartFcn=sigbuilder_block('start');  StopFcn=sigbuilder_block('stop');  ClipboardFcn=sigbuilder_block('clipboard');  mask(Sigbuilder block){tuvar=[0:10]}
      mask help: Simulink:masks:SigbuilderBlock_MD
      mask init:
      | if ~strcmp(get_param(bdroot(gcbh),'SimulationStatus'),'stopped') tuvar = sigbuilder_block('maskInit'); end
      settings: CopyFcn=sigbuilder_block('copy');  DeleteFcn=sigbuilder_block('delete');  ModelCloseFcn=sigbuilder_block('modelClose');  PreSaveFcn=sigbuilder_block('preSave');  PauseFcn=sigbuilder_block('pause');  ContinueFcn=sigbuilder_block('continue');  NameChangeFcn=sigbuilder_block('namechange');  OpenFcn=sigbuilder_block('open',[437.6 199.2 550.4 400 ]);  CloseFcn=sigbuilder_block('close');
      mask Display: plot(0, 0, 100, 100,[2, 2, 32, 32, 2], [68, 8, 8, 68, 68],[32, 2], [38, 38], [32, 19, 2],[53, 60, 44], [32, 17, 17, 2],[16, 16, 31, 31]);txt = getActiveGroup(gcbh);text(2, 100, txt,'verticalAlignment', 'top');
  Simulink-PS Converter : nesl_utility/Simulink-PS Converter  PhysicalDomain=network_engine_domain  SubClassName=ps_input  LeftPortType=input  RightPortType=output  PseudoPeriodic=off  Frequencies=[]  NoiseDistribution=none  NoiseParameters=[]  Unit=1  AffineConversion=off  FilteringAndDerivatives=provide  SimscapeFilterOrder=1  InputFilterTimeConstant=0.001  UdotUserProvided=0
  Simulink-PS Converter1 : nesl_utility/Simulink-PS Converter  PhysicalDomain=network_engine_domain  SubClassName=ps_input  LeftPortType=input  RightPortType=output  PseudoPeriodic=off  Frequencies=[]  NoiseDistribution=none  NoiseParameters=[]  Unit=1  AffineConversion=off  FilteringAndDerivatives=provide  SimscapeFilterOrder=1  InputFilterTimeConstant=0.001  UdotUserProvided=0
  Simulink-PS Converter2 : nesl_utility/Simulink-PS Converter  PhysicalDomain=network_engine_domain  SubClassName=ps_input  LeftPortType=input  RightPortType=output  PseudoPeriodic=off  Frequencies=[]  NoiseDistribution=none  NoiseParameters=[]  Unit=1  AffineConversion=off  FilteringAndDerivatives=provide  SimscapeFilterOrder=1  InputFilterTimeConstant=0.001  UdotUserProvided=0
  Simulink-PS Converter3 : nesl_utility/Simulink-PS Converter  Commented=on  PhysicalDomain=network_engine_domain  SubClassName=ps_input  LeftPortType=input  RightPortType=output  PseudoPeriodic=off  Frequencies=[]  NoiseDistribution=none  NoiseParameters=[]  Unit=1  AffineConversion=off  FilteringAndDerivatives=provide  SimscapeFilterOrder=1  InputFilterTimeConstant=0.001  UdotUserProvided=0
  Simulink-PS Converter4 : nesl_utility/Simulink-PS Converter  Commented=on  PhysicalDomain=network_engine_domain  SubClassName=ps_input  LeftPortType=input  RightPortType=output  PseudoPeriodic=off  Frequencies=[]  NoiseDistribution=none  NoiseParameters=[]  Unit=1  AffineConversion=off  FilteringAndDerivatives=provide  SimscapeFilterOrder=1  InputFilterTimeConstant=0.001  UdotUserProvided=0
  Simulink-PS Converter5 : nesl_utility/Simulink-PS Converter  Commented=on  PhysicalDomain=network_engine_domain  SubClassName=ps_input  LeftPortType=input  RightPortType=output  PseudoPeriodic=off  Frequencies=[]  NoiseDistribution=none  NoiseParameters=[]  Unit=1  AffineConversion=off  FilteringAndDerivatives=provide  SimscapeFilterOrder=1  InputFilterTimeConstant=0.001  UdotUserProvided=0
  Single-Acting Hydraulic Cylinder (Simple)2 : sh_lib/Hydraulic Cylinders/Single-Acting Hydraulic Cylinder (Simple)  Commented=on  area=0.001 m^2  stroke=0.5 m  init_pos=0 m  penetr_coeff=1e12 s*N/m^2  or=1
      settings: InternalSimscapePortConfiguration="{\"Bottom\":[],\"Left\":[{\"id\":\"C\",\"label\":\"C\",\"type\":\"foundation.mechanical.translational.translational\"},{\"id\":\"A\",\"label\":\"A\",\"type\":\"foundation.hydraulic.hydraulic\"}],\"Right\":[{\"id\":\"R\",\"label\":\"R\",\"type\":\"foundation.mechanical.translational.translational\"},{\"id\":\"P\",\"label\":\"P\",\"type\":\"output\"}],\"Top\":[]}"
  Single-Acting Hydraulic Cylinder (Simple)3 : sh_lib/Hydraulic Cylinders/Single-Acting Hydraulic Cylinder (Simple)  Commented=on  area=0.001 m^2  stroke=0.5 m  init_pos=0 m  penetr_coeff=1e12 s*N/m^2  or=1
      settings: InternalSimscapePortConfiguration="{\"Bottom\":[],\"Left\":[{\"id\":\"C\",\"label\":\"C\",\"type\":\"foundation.mechanical.translational.translational\"},{\"id\":\"A\",\"label\":\"A\",\"type\":\"foundation.hydraulic.hydraulic\"}],\"Right\":[{\"id\":\"R\",\"label\":\"R\",\"type\":\"foundation.mechanical.translational.translational\"},{\"id\":\"P\",\"label\":\"P\",\"type\":\"output\"}],\"Top\":[]}"
  Solver Configuration : nesl_utility/Solver Configuration  PhysicalDomain=network_engine_domain  SubClassName=solver  LeftPortType=input  RightPortType=generic  Tones=[]  Harmonics=[]  SimulateNoise=off  Profile=off  UseLocalSampling=off  EnableSwitchedLinearOptims=on  FrequencyDomain=off  UseCCode=off  RelTol=0.001  AbsTol=1e-06  MinStep=1e-09  ToWorkspace=off  RevertToSquareIcSolve=off  NumHomotopyIterations=100  PhasorMode=off  PhasorModeNumHarmonics=1  ConsistencySolver=NEWTON_FTOL  IndexReductionMethod=DerivativeReplacement  DoDC=off  ResidualTolerance=1e-09  ConsistencyTolSource=GLOBAL  ConsistencyAbsTol=0.001  ConsistencyRelTol=0.001  ConsistencyTolFactor=0.001  UseLocalSolver=off  LocalSolverChoice=NE_BACKWARD_EULER_ADVANCER  ResolveIndetEquations=on  FunctionEvalNumThread=1  LocalSolverSampleTime=0.001  DoFixedCost=off  MaxNonlinIter=3  MaxModeIter=2  ComputeImpulses=off  ImpulseIterations=2  LinearAlgebra=auto  LinearAlgebraNumThread=0  EquationFormulation=NE_TIME_EF  DelaysMemoryBudget=1024  AutomaticFiltering=on  FilteringTimeConstant=0.001  PartitionStorageMethod=AS_NEEDED  PartitionMemoryBudget=1024  PartitionMethod=ROBUST  MultibodyUseLocalSolver=off  MultibodyLocalSolverChoice=ODE1  MultibodyLocalSolverSampleTime=0.001
  Solver Configuration2 : nesl_utility/Solver Configuration  Commented=on  PhysicalDomain=network_engine_domain  SubClassName=solver  LeftPortType=input  RightPortType=generic  Tones=[]  Harmonics=[]  SimulateNoise=off  Profile=off  UseLocalSampling=off  EnableSwitchedLinearOptims=on  FrequencyDomain=off  UseCCode=off  RelTol=0.001  AbsTol=1e-06  MinStep=1e-09  ToWorkspace=off  RevertToSquareIcSolve=off  NumHomotopyIterations=100  PhasorMode=off  PhasorModeNumHarmonics=1  ConsistencySolver=NEWTON_FTOL  IndexReductionMethod=DerivativeReplacement  DoDC=off  ResidualTolerance=1e-09  ConsistencyTolSource=GLOBAL  ConsistencyAbsTol=0.001  ConsistencyRelTol=0.001  ConsistencyTolFactor=0.001  UseLocalSolver=off  LocalSolverChoice=NE_BACKWARD_EULER_ADVANCER  ResolveIndetEquations=on  FunctionEvalNumThread=1  LocalSolverSampleTime=0.001  DoFixedCost=off  MaxNonlinIter=3  MaxModeIter=2  ComputeImpulses=off  ImpulseIterations=2  LinearAlgebra=auto  LinearAlgebraNumThread=0  EquationFormulation=NE_TIME_EF  DelaysMemoryBudget=1024  AutomaticFiltering=on  FilteringTimeConstant=0.001  PartitionStorageMethod=AS_NEEDED  PartitionMemoryBudget=1024  PartitionMethod=ROBUST  MultibodyUseLocalSolver=off  MultibodyLocalSolverChoice=ODE1  MultibodyLocalSolverSampleTime=0.001
  Solver Configuration3 : nesl_utility/Solver Configuration  Commented=on  PhysicalDomain=network_engine_domain  SubClassName=solver  LeftPortType=input  RightPortType=generic  Tones=[]  Harmonics=[]  SimulateNoise=off  Profile=off  UseLocalSampling=off  EnableSwitchedLinearOptims=on  FrequencyDomain=off  UseCCode=off  RelTol=0.001  AbsTol=1e-06  MinStep=1e-09  ToWorkspace=off  RevertToSquareIcSolve=off  NumHomotopyIterations=100  PhasorMode=off  PhasorModeNumHarmonics=1  ConsistencySolver=NEWTON_FTOL  IndexReductionMethod=DerivativeReplacement  DoDC=off  ResidualTolerance=1e-09  ConsistencyTolSource=GLOBAL  ConsistencyAbsTol=0.001  ConsistencyRelTol=0.001  ConsistencyTolFactor=0.001  UseLocalSolver=off  LocalSolverChoice=NE_BACKWARD_EULER_ADVANCER  ResolveIndetEquations=on  FunctionEvalNumThread=1  LocalSolverSampleTime=0.001  DoFixedCost=off  MaxNonlinIter=3  MaxModeIter=2  ComputeImpulses=off  ImpulseIterations=2  LinearAlgebra=auto  LinearAlgebraNumThread=0  EquationFormulation=NE_TIME_EF  DelaysMemoryBudget=1024  AutomaticFiltering=on  FilteringTimeConstant=0.001  PartitionStorageMethod=AS_NEEDED  PartitionMemoryBudget=1024  PartitionMethod=ROBUST  MultibodyUseLocalSolver=off  MultibodyLocalSolverChoice=ODE1  MultibodyLocalSolverSampleTime=0.001
  Step1 : Step  Commented=on  SampleTime=0
  Step2 : Step  SampleTime=1
  Sum : Sum  Inputs=|++
  Translational Damper : fl_lib/Mechanical/Translational Elements/Translational Damper  D=800 N/(m/s)  v_specify=off  v_priority=None  v=0 m/s  v_nominal_specify=off  v_nominal_unit=m/s  v_nominal_value=1  f_specify=off  f_priority=None  f=0 N  f_nominal_specify=off  f_nominal_unit=N  f_nominal_value=1
  Translational Damper1 : fl_lib/Mechanical/Translational Elements/Translational Damper  D=800 N/(m/s)  v_specify=off  v_priority=None  v=0 m/s  v_nominal_specify=off  v_nominal_unit=m/s  v_nominal_value=1  f_specify=off  f_priority=None  f=0 N  f_nominal_specify=off  f_nominal_unit=N  f_nominal_value=1
  Translational Spring2 : fl_lib/Mechanical/Translational Elements/Translational Spring  Commented=on  spr_rate=50000 N/m  v_specify=off  v_priority=None  v=0 m/s  v_nominal_specify=off  v_nominal_unit=m/s  v_nominal_value=1  f_specify=off  f_priority=None  f=0 N  f_nominal_specify=off  f_nominal_unit=N  f_nominal_value=1  x_specify=off  x_priority=High  x=0 m  x_nominal_specify=off  x_nominal_unit=m  x_nominal_value=1
  Variable Orifice1 : sh_lib/Orifices/Variable Orifice  Commented=on  mdl_type=1  area_max=1e-4 m^2  opening_max=2e-4 m  opening_tab=[-.002, 0, .002, .005, .015] m  area_tab=[1e-09, 2.0352e-07, 4.0736e-05, .00011438, .00034356] m^2  pressure_tab=[-10000000, -5000000, -2000000, 2000000, 5000000, 10000000] Pa  flow_rate_tab=[-1e-07, -7.0711e-08, -4.4721e-08, 4.4721e-08, 7.0711e-08, 1e-07; -2.0352e-05, -1.4391e-05, -9.1017e-06, 9.1017e-06, 1.4391e-05, 2.0352e-05; -.0040736, -.0028805, -.0018218, .0018218, .0028805, .0040736; -.011438, -.0080879, -.0051152, .0051152, .0080879, .011438; -.034356, -.024293, -.015364, .015364, .024293, .034356] m^3/s  interp_method=1  extrap_method=1  or=1  C_d=0.61  x_0=0 m  A_leak=1e-12 m^2  lam_spec=1  B_lam=0.999  Re_cr=12  flow_rate_specify=off  flow_rate_priority=None  flow_rate=0 m^3/s  flow_rate_nominal_specify=off  flow_rate_nominal_unit=m^3/s  flow_rate_nominal_value=1  pressure_drop_specify=off  pressure_drop_priority=None  pressure_drop=0 Pa  pressure_drop_nominal_specify=off  pressure_drop_nominal_unit=Pa  pressure_drop_nominal_value=1
      settings: InternalSimscapePortConfiguration="{\"Bottom\":[],\"Left\":[{\"id\":\"S\",\"label\":\"S\",\"type\":\"input\"},{\"id\":\"A\",\"label\":\"A\",\"type\":\"foundation.hydraulic.hydraulic\"}],\"Right\":[{\"id\":\"B\",\"label\":\"B\",\"type\":\"foundation.hydraulic.hydraulic\"}],\"Top\":[]}"
  wires:
  PS-Simulink Converter4/1 -> Scope2/1
  Constant/1 -> Simulink-PS Converter2/1
  ? -> Sum/2
  Pulse Generator1/1 -> Simulink-PS Converter3/1
  PS-Simulink Converter13/1 -> Scope4/1  "x1"
  Constant1/1 -> Simulink-PS Converter5/1
  Gain1/1 -> Simulink-PS Converter4/1
  Clock1/1 -> Gain1/1
  PS-Simulink Converter8/1 -> Scope5/3  "p1"
  PS-Simulink Converter12/1 -> Scope7/1  "x"
  PS-Simulink Converter11/1 -> Scope6/1
  PS-Simulink Converter7/1 -> Scope4/2  "x"
  PS-Simulink Converter9/1 -> Scope5/2  "p2"
  PS-Simulink Converter10/1 -> Scope5/1  "p3"
  PS-Simulink Converter14/1 -> Scope8/1  "x"
  Constant2/1 -> Sum/1
  Sum/1 -> Simulink-PS Converter/1, Scope/1
  PS-Simulink Converter1/1 -> Scope1/1
  PS-Simulink Converter2/1 -> Scope3/1  "x"
  connections:
  Hydraulic Reference/LConn1 -- 4-Way Directional Valve/RConn3 -- Hydraulic Pressure Sensor/RConn1 -- Pressure Relief Valve/RConn1 -- Hydraulic Constant Flow Rate Source2/RConn1 -- Solver Configuration/RConn1 -- Hydraulic Fluid/RConn1
  Double-Acting Hydraulic Cylinder (Simple)/LConn2 -- Hydraulic Pipeline/RConn1
  Hydraulic Flow Rate Sensor/RConn1 -- PS-Simulink Converter4/LConn1
  Pressure Relief Valve/LConn1 -- Hydraulic Pressure Sensor/LConn1 -- 4-Way Directional Valve/RConn2 -- Hydraulic Constant Flow Rate Source2/LConn1
  4-Way Directional Valve/LConn1 -- Hydraulic Flow Rate Sensor/LConn1
  Ideal Force Source/RConn1 -- Simulink-PS Converter2/RConn1
  4-Way Directional Valve/RConn1 -- Simulink-PS Converter/RConn1
  Single-Acting Hydraulic Cylinder (Simple)3/RConn1 -- Ideal Force Source1/RConn2 -- Mass1/LConn1
  Hydraulic Constant Flow Rate Source1/RConn1 -- 3-Way Directional Valve1/RConn3 -- Hydraulic Pressure Sensor5/RConn1 -- Hydraulic Pressure Sensor4/RConn1 -- Fixed Orifice2/RConn1 -- Hydraulic Pressure Sensor3/RConn1 -- Pressure Relief Valve1/RConn1 -- Hydraulic Reference1/LConn1 -- Hydraulic Fluid1/RConn1 -- Solver Configuration2/RConn1
  Hydraulic Constant Flow Rate Source1/LConn1 -- Pressure Relief Valve1/LConn1 -- 3-Way Directional Valve1/RConn2
  Hydraulic Pressure Sensor3/LConn1 -- Fixed Orifice2/LConn1 -- Variable Orifice1/LConn2 -- Hydraulic Flow Rate Sensor1/RConn2
  Hydraulic Pressure Sensor4/LConn1 -- Fixed Orifice3/LConn1 -- Variable Orifice1/RConn1
  Solver Configuration3/RConn1 -- Ideal Force Sensor1/RConn1 -- Mechanical Translational Reference8/LConn1
  Single-Acting Hydraulic Cylinder (Simple)2/LConn2 -- Single-Acting Hydraulic Cylinder (Simple)3/LConn2 -- Fixed Orifice3/RConn1 -- Hydraulic Pressure Sensor5/LConn1
  Ideal Force Source1/LConn1 -- Mechanical Translational Reference9/LConn1
  Single-Acting Hydraulic Cylinder (Simple)2/RConn1 -- Translational Spring2/RConn1
  Hydraulic Pressure Sensor3/RConn2 -- PS-Simulink Converter8/LConn1
  Ideal Force Sensor1/RConn2 -- PS-Simulink Converter12/LConn1
  Hydraulic Flow Rate Sensor1/RConn1 -- PS-Simulink Converter11/LConn1
  Mechanical Translational Reference11/LConn1 -- Single-Acting Hydraulic Cylinder (Simple)3/LConn1
  Mechanical Translational Reference7/LConn1 -- Single-Acting Hydraulic Cylinder (Simple)2/LConn1
  PS-Simulink Converter10/LConn1 -- Hydraulic Pressure Sensor5/RConn2
  3-Way Directional Valve1/LConn1 -- Hydraulic Flow Rate Sensor1/LConn1
  PS-Simulink Converter7/LConn1 -- Single-Acting Hydraulic Cylinder (Simple)2/RConn2
  Ideal Force Source1/RConn1 -- Simulink-PS Converter5/RConn1
  PS-Simulink Converter9/LConn1 -- Hydraulic Pressure Sensor4/RConn2
  PS-Simulink Converter13/LConn1 -- Single-Acting Hydraulic Cylinder (Simple)3/RConn2
  Simulink-PS Converter3/RConn1 -- 3-Way Directional Valve1/RConn1
  Simulink-PS Converter4/RConn1 -- Variable Orifice1/LConn1
  Translational Spring2/LConn1 -- Mechanical Translational Reference6/LConn1
  Double-Acting Hydraulic Cylinder (Simple)/RConn2 -- Hydraulic Pipeline1/LConn1
  Double-Acting Hydraulic Cylinder (Simple)/LConn1 -- Mechanical Translational Reference1/LConn1
  Mass2/LConn1 -- Double-Acting Hydraulic Cylinder (Simple)/RConn1 -- Ideal Force Source/RConn2 -- Translational Damper/LConn1 -- Ideal Translational Motion Sensor1/LConn1
  Translational Damper/RConn1 -- Ideal Translational Motion Sensor1/RConn1 -- Mechanical Translational Reference/LConn1
  Ideal Translational Motion Sensor1/RConn3 -- PS-Simulink Converter14/LConn1
  PS-Simulink Converter1/LConn1 -- Hydraulic Pressure Sensor/RConn2
  PS-Simulink Converter2/LConn1 -- Ideal Translational Motion Sensor1/RConn2
  Hydraulic Pipeline/LConn1 -- Hydraulic Flow Rate Sensor/RConn2
  Hydraulic Pipeline1/RConn1 -- 4-Way Directional Valve/LConn2
  Ideal Force Source/LConn1 -- Mechanical Translational Reference3/LConn1

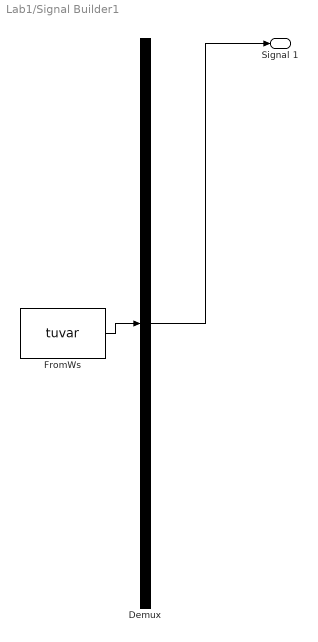
== system Lab1/Signal Builder1 ==
  Demux : Demux  Tag=STV Demux  Outputs=1
      settings: DisplayOption=none
  FromWs : FromWorkspace  Tag=STV FromWs  VariableName=tuvar
      SigBuilderData=|
      | common.afterFinalStr = 'Extrapolate'
      | common.sampleTime = 0
      | dataSet.timeRange = [0 10]
      | dataSet.name = 'Group 1'
      | sbobj.Groups.Name = 'Group 1'
      | sbobj.Groups.Signals.Name = 'Signal 1'
      | sbobj.Groups.Signals.XData = [0 4 4 6 6 10]
      | sbobj.Groups.Signals.YData = [0 0 1 1 0 0]
  Signal 1 : Outport  Tag=STV Outport
  wires:
  Demux/1 -> Signal 1/1
  FromWs/1 -> Demux/1
